simulink model "MackeyGlass"  (R2014b)
settings: Solver=ode45  StartTime=0.0  StopTime=10.0  RelTol=1e-3
values from neighbouring files (symbols this model uses):
  b = 0.7    [Run_Aizawa.m]    (also in Run_Arneodo.m = 3.5; Run_Chen.m = 3; Run_Chua.m = 28; Run_Duffing.m = 100)
  n = 10    [Run_MackeyGlass.m]
  tau = 5    [Run_MackeyGlass.m]
  y = 1    [Run_Duffing.m]    (also in Run_MackeyGlass.m)
undefined symbols (not defined in the file or in its folder): param
settings Model: Creator=Arek  LastModifiedBy=Arek

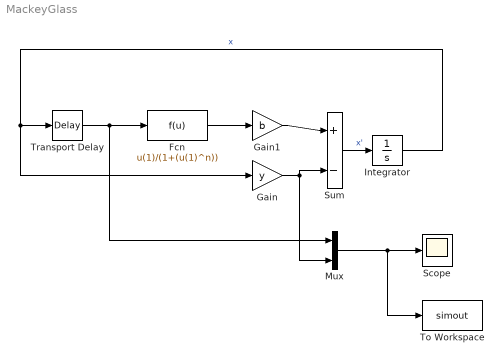
== system MackeyGlass ==
  Fcn : Fcn  Expr=u(1)/(1+(u(1)^n))
  Gain : Gain  Gain=y
  Gain1 : Gain  Gain=b
  Integrator : Integrator  InitialCondition=param.ic
  Mux : Mux  Inputs=2
  Scope : Scope
  Sum : Sum  Inputs=+|-
  To Workspace : ToWorkspace  VariableName=simout  SaveFormat=Timeseries  SampleTime=-1
  Transport Delay : TransportDelay  DelayTime=tau  BufferSize=4096
  wires:
  Sum/1 -> Integrator/1  "x'"
  Gain/1 -> Mux/2, Sum/2
  Integrator/1 -> Transport Delay/1, Gain/1  "x"
  Transport Delay/1 -> Fcn/1, Mux/1
  Mux/1 -> To Workspace/1, Scope/1
  Gain1/1 -> Sum/1
  Fcn/1 -> Gain1/1
